simulink model "SingleAgent_Model"  (R2017b)
settings: Solver=VariableStepAuto  StartTime=0.0  StopTime=10.0  RelTol=1e-3
values from neighbouring files (symbols this model uses):
  p02 = zeros(SInfo2.n, 1)    [Parameters.m]
  q01 = zeros(SInfo1.n, 1)    [Parameters.m]
undefined symbols (not defined in the file or in its folder): p0, q0
settings Model: Creator=oscar  LastModifiedBy=oscar

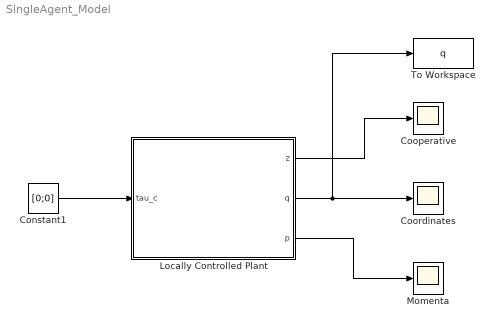
== system SingleAgent_Model ==
  Constant1 : Constant  Value=[0;0]
  Cooperative : Scope
  Coordinates : Scope
  Locally Controlled Plant : Subsystem
  Momenta : Scope
  To Workspace : ToWorkspace  VariableName=q  SaveFormat=Timeseries  SampleTime=-1
  wires:
  Locally Controlled Plant/2(q) -> To Workspace/1, Coordinates/1
  Locally Controlled Plant/3(p) -> Momenta/1
  Constant1/1 -> Locally Controlled Plant/1(tau_c)
  Locally Controlled Plant/1(z) -> Cooperative/1

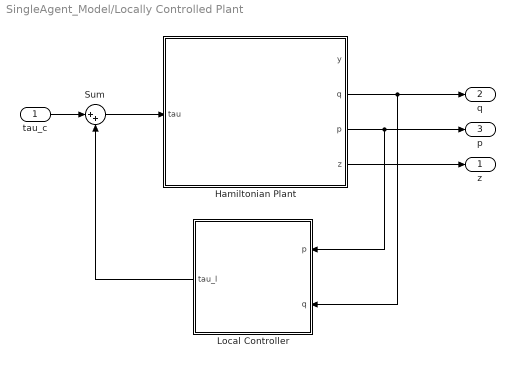
== system SingleAgent_Model/Locally Controlled Plant ==
  tau_c : Inport
  Hamiltonian Plant : Subsystem
  Local Controller : Subsystem
  Sum : Sum  Inputs=|++
  z : Outport
  q : Outport  Port=2
  p : Outport  Port=3
  wires:
  Sum/1 -> Hamiltonian Plant/1(tau)
  Local Controller/1(tau_l) -> Sum/2
  tau_c/1 -> Sum/1
  Hamiltonian Plant/3(p) -> p/1, Local Controller/1(p)
  Hamiltonian Plant/2(q) -> q/1, Local Controller/2(q)
  Hamiltonian Plant/4(z) -> z/1

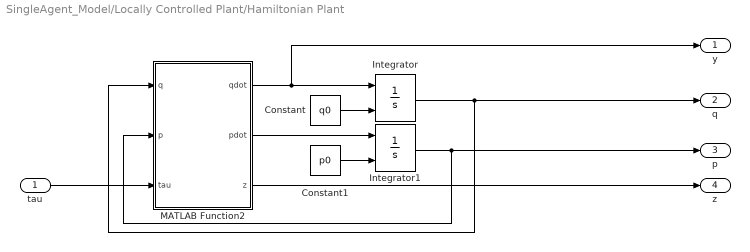
== system SingleAgent_Model/Locally Controlled Plant/Hamiltonian Plant ==
  tau : Inport
  Constant : Constant  Value=q0
  Constant1 : Constant  Value=p0
  Integrator : Integrator  InitialConditionSource=external  InitialCondition=q01
  Integrator1 : Integrator  InitialConditionSource=external  InitialCondition=p02
  MATLAB Function2 : MATLAB Function  TreatAsAtomicUnit=on
  y : Outport
  q : Outport  Port=2
  p : Outport  Port=3
  z : Outport  Port=4
  wires:
  tau/1 -> MATLAB Function2/3(tau)
  MATLAB Function2/2(pdot) -> Integrator1/1
  Integrator1/1 -> MATLAB Function2/2(p), p/1
  Integrator/1 -> MATLAB Function2/1(q), q/1
  MATLAB Function2/1(qdot) -> y/1, Integrator/1
  Constant/1 -> Integrator/2
  Constant1/1 -> Integrator1/2
  MATLAB Function2/3(z) -> z/1

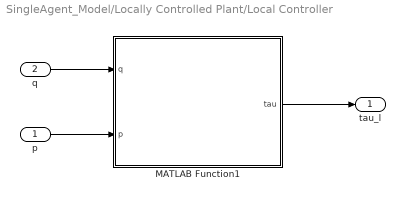
== system SingleAgent_Model/Locally Controlled Plant/Local Controller ==
  p : Inport
  q : Inport  Port=2
  MATLAB Function1 : MATLAB Function  TreatAsAtomicUnit=on
  tau_l : Outport
  wires:
  q/1 -> MATLAB Function1/1(q)
  p/1 -> MATLAB Function1/2(p)
  MATLAB Function1/1(tau) -> tau_l/1

== matlab function SingleAgent_Model/Locally Controlled Plant/Hamiltonian Plant/MATLAB Function2 ==
  data: q input; qdot output; p input; tau input; pdot output; z output
function [qdot, pdot, z] = fcn(q, p, tau)

    coder.extrinsic('M_point_mass');
    qdot = zeros(2, 1);
    pdot = zeros(2, 1);
    z = 0;
    [qdot, pdot, z] = M_point_mass(q, p, tau);

== matlab function SingleAgent_Model/Locally Controlled Plant/Local Controller/MATLAB Function1 ==
  data: q input; tau output; p input
function tau = LocalControl(q, p)
    

coder.extrinsic('LC_point_mass');
tau = zeros(2, 1);
tau = LC_point_mass(q, p);
